simulink model "PID_PI_LADRC"  (R2021a)
settings: Solver=VariableStepAuto  StartTime=0.0  StopTime=Tsim  RelTol=1e-3
undefined symbols (not defined in the file or in its folder): Ac, Alpha, Bc, Cc, Cg, Kconva, Kconvp, Krad, L, mcecool, mcehot, mcerad, n, Rp, Tamb, Vfan, zo
libraries: pid_lib x1
settings Model: Creator=djah0  LastModifiedBy=djah0
settings DataIOCC: ReturnWorkspaceOutputs=off

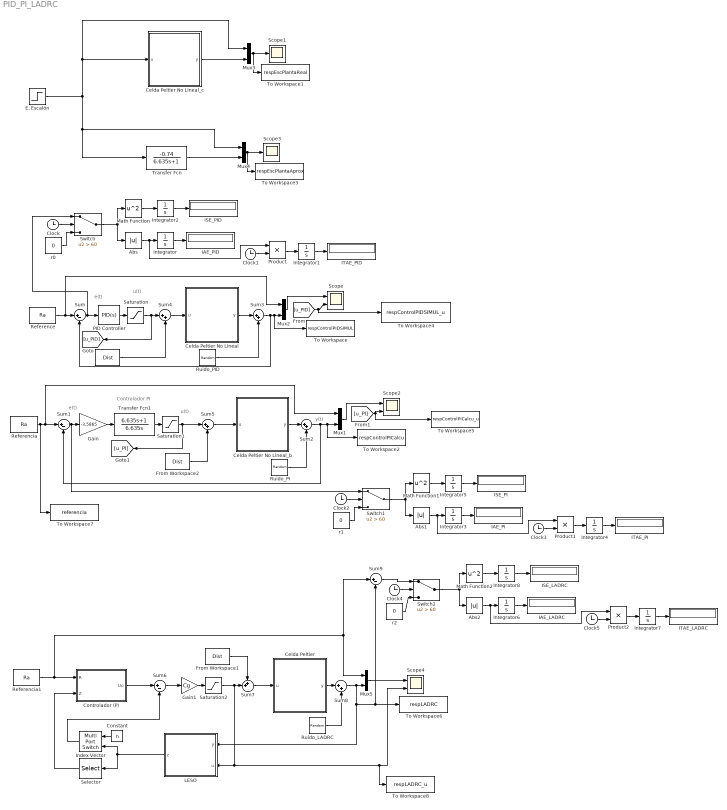
== system PID_PI_LADRC ==
  note: Controlador PI
  note: e(t)
  note: y(t)
  note: u(t)
  note: e(t)
  note: u(t)
  " " : FromWorkspace  VariableName=Dist
  Abs : Abs
  Abs1 : Abs
  Abs2 : Abs
  Celda Peltier : Subsystem
  Celda Peltier No Lineal : Subsystem
  Celda Peltier No Lineal_b : Subsystem
  Celda Peltier No Lineal_c : Subsystem
  Clock{,1..5} (6 alike) : Clock
  Constant : Constant  Value=n
  Controlador (P) : Subsystem
  E. Escalón : Step  Time=0  After=26  SampleTime=0
  From Workspace1 : FromWorkspace  VariableName=Dist
  From Workspace2 : FromWorkspace  VariableName=Dist
  Gain : Gain  Gain=-3.5865
  Gain1 : Gain  Gain=Cg
  IAE_LADRC : Display
  IAE_PI : Display
  IAE_PID : Display
  ISE_LADRC : Display
  ISE_PI : Display
  ISE_PID : Display
  ITAE_LADRC : Display
  ITAE_PI : Display
  ITAE_PID : Display
  Index Vector : MultiPortSwitch  Inputs=1
  Integrator{,1..8} (9 alike) : Integrator
  LESO : Subsystem
  Math Function : Math  Operator=square  SaturateOnIntegerOverflow=on
  Math Function1 : Math  Operator=square  SaturateOnIntegerOverflow=on
  Math Function2 : Math  Operator=square  SaturateOnIntegerOverflow=on
  Mux{1..5} (5 alike) : Mux  Inputs=2
  PID Controller : pid_lib/PID Controller  Controller=PID  Form=Parallel  TimeDomain=Continuous-time  UseExternalTs=off  SampleTime=-1  IntegratorMethod=Forward Euler  FilterMethod=Forward Euler  ControllerParametersSource=internal  P=-7.59310160847849  I=-3.05370465594005  D=0.689315335908169  UseFilter=on  N=11.0154253255872  TunerSelectOption=Transfer Function Based (PID Tuner App)  InitialConditionSource=internal  InitialConditionForIntegrator=26  InitialConditionForFilter=0  DifferentiatorICPrevScaledInput=0  ExternalReset=none  TrackingMode=off  Kt=1  LimitOutput=off  SatLimitsSource=internal  UpperSaturationLimit=inf  LowerSaturationLimit=-inf  LinearizeAsGain=on  AntiWindupMode=none  Kb=1  POutMin=[]  POutMax=[]  IOutMin=[]  IOutMax=[]  DOutMin=[]  DOutMax=[]  NOutMin=[]  NOutMax=[]  SumOutMin=[]  SumOutMax=[]  SaturationOutMin=[]  SaturationOutMax=[]  PParamMin=[]  PParamMax=[]  IParamMin=[]  IParamMax=[]  DParamMin=[]  DParamMax=[]  NParamMin=[]  NParamMax=[]  KbParamMin=[]  KbParamMax=[]  KtParamMin=[]  KtParamMax=[]  KbOutMin=[]  KbOutMax=[]  KtOutMin=[]  KtOutMax=[]  IntegratorOutMin=[]  IntegratorOutMax=[]  FilterOutMin=[]  FilterOutMax=[]  SumI1OutMin=[]  SumI1OutMax=[]  SumI2OutMin=[]  SumI2OutMax=[]  SumI3OutMin=[]  SumI3OutMax=[]  SumI4OutMin=[]  SumI4OutMax=[]  SumDOutMin=[]  SumDOutMax=[]  DifferentiatorOutMin=[]  DifferentiatorOutMax=[]  FilterDiffOutCoefMin=[]  FilterDiffOutCoefMax=[]  ReciprocalOutMin=[]  ReciprocalOutMax=[]  SumDenOutMin=[]  SumDenOutMax=[]  SumNumOutMin=[]  SumNumOutMax=[]  DivideOutMin=[]  DivideOutMax=[]  UdiffTsProdOutMin=[]  UdiffTsProdOutMax=[]  NTsProdOutMin=[]  NTsProdOutMax=[]  UintegralTsProdOutMin=[]  UintegralTsProdOutMax=[]  UngainTsProdOutMin=[]  UngainTsProdOutMax=[]  IntegratorContinuousStateAttributes=''  IntegratorStateMustResolveToSignalObject=off  IntegratorRTWStateStorageClass=Auto  FilterContinuousStateAttributes=''  FilterStateMustResolveToSignalObject=off  FilterRTWStateStorageClass=Auto  ParallelPVariant=InternalParameters  IdealPVariant=Disabled  IVariant=InternalParameters  DVariant=InternalParameters  IntegratorVariant=Continuous  SatVariant=Disabled  AWVariant=Passthrough  PCopyVariant=Disabled  TRVariant=Disabled  FdbkBlocksVariant=Forward  IdealPFdbkVariant=Disabled  SatFdbkVariant=Disabled  DerivativeFilterVariant=ContFilter  NVariant=InternalParameters  NCopyVariant=Disabled  FilterICVariant=InternalICsFilter  IntegratorICVariant=InternalICs  ExternalResetVariant=Disabled  TRSumVariant=Passthrough  SumFdbkVariant=Disabled  SumVariant=Sum_PID  TsampFilterVariant=InternalTs  TsampNgainVariant=Passthrough  TsampIntegralVariant=Passthrough  ExternalSaturationOutDataTypeStr=Inherit: Same as second input
  Product : Product
  Product1 : Product
  Product2 : Product
  Reference : FromWorkspace  VariableName=Ra
  Referencia : FromWorkspace  VariableName=Ra
  Referencia1 : FromWorkspace  VariableName=Ra
  Ruido_LADRC : RandomNumber  Variance=0.002  SampleTime=0.2
  Ruido_PI : RandomNumber  Variance=0.002  SampleTime=0.2
  Ruido_PID : RandomNumber  Variance=0.002  SampleTime=0.2
  Saturation : Saturate  UpperLimit=100  LowerLimit=0
  Saturation1 : Saturate  UpperLimit=100  LowerLimit=0
  Saturation2 : Saturate  UpperLimit=100  LowerLimit=0
  Scope : Scope  NumInputPorts=2
  Scope1 : Scope
  Scope2 : Scope  NumInputPorts=2
  Scope3 : Scope
  Scope4 : Scope  NumInputPorts=2
  Selector : Selector  InputPortWidth=n  IndexOptions=Index vector (dialog)  Indices=1:n-1  OutputSizes=1
  Sum{,1,6,9} (4 alike) : Sum  Inputs=|+-
  Sum{2..5,8} (5 alike) : Sum  Inputs=|++
  Sum7 : Sum  Inputs=++|
  Switch : Switch  Criteria=u2 > Threshold  Threshold=60
  Switch1 : Switch  Criteria=u2 > Threshold  Threshold=60
  Switch2 : Switch  Criteria=u2 > Threshold  Threshold=60
  To Workspace : ToWorkspace  VariableName=respControlPIDSIMUL  SaveFormat=Timeseries  SampleTime=-1
  To Workspace1 : ToWorkspace  VariableName=respEscPlantaReal  SaveFormat=Timeseries  SampleTime=-1
  To Workspace2 : ToWorkspace  VariableName=respControlPICalcu  SaveFormat=Timeseries  SampleTime=-1
  To Workspace3 : ToWorkspace  VariableName=respEscPlantaAprox  SaveFormat=Timeseries  SampleTime=-1
  To Workspace4 : ToWorkspace  VariableName=respControlPIDSIMUL_u  SaveFormat=Timeseries  SampleTime=-1
  To Workspace5 : ToWorkspace  VariableName=respControlPICalcu_u  SaveFormat=Timeseries  SampleTime=-1
  To Workspace6 : ToWorkspace  VariableName=respLADRC  SaveFormat=Timeseries  SampleTime=-1
  To Workspace7 : ToWorkspace  VariableName=referencia  SaveFormat=Timeseries  SampleTime=-1
  To Workspace8 : ToWorkspace  VariableName=respLADRC_u  SaveFormat=Timeseries  SampleTime=-1
  Transfer Fcn : TransferFcn  Numerator=[-0.74]  Denominator=[6.635 1]
  Transfer Fcn1 : TransferFcn  Numerator=[6.635 1]  Denominator=[6.635 0]
  r0 : Constant  Value=0
  r1 : Constant  Value=0
  r2 : Constant  Value=0
  wires:
  Mux2/1 -> Scope/1
  Reference/1 -> Mux2/1, Sum/1
  Referencia/1 -> To Workspace7/1, Mux1/1, Sum1/1
  Sum1/1 -> Switch1/1, Gain/1
  Mux1/1 -> Scope2/1
  Gain/1 -> Transfer Fcn1/1
  Sum/1 -> Switch/1, PID Controller/1
  Sum2/1 -> Sum1/2, To Workspace2/1, Mux1/2
  Sum3/1 -> Sum/2, To Workspace/1, Mux2/2
  [u_PID] -> To Workspace4/1, Scope/2
  [u_PI] -> To Workspace5/1, Scope2/2
  PID Controller/1 -> Saturation/1
  Transfer Fcn1/1 -> Saturation1/1
  Saturation1/1 -> Sum5/1, [u_PI]
  Saturation/1 -> [u_PID], Sum4/1
  Sum4/1 -> Celda Peltier No Lineal/1(u)
  " "/1 -> Sum4/2
  Celda Peltier No Lineal/1(y) -> Sum3/1
  Celda Peltier No Lineal_b/1(y) -> Sum2/1
  Sum5/1 -> Celda Peltier No Lineal_b/1(u)
  From Workspace2/1 -> Sum5/2
  Abs/1 -> Product/1, Integrator/1
  Integrator/1 -> IAE_PID/1
  r0/1 -> Switch/3
  Clock/1 -> Switch/2
  Switch/1 -> Math Function/1, Abs/1
  Math Function/1 -> Integrator2/1
  Integrator2/1 -> ISE_PID/1
  Clock1/1 -> Product/2
  Product/1 -> Integrator1/1
  Integrator1/1 -> ITAE_PID/1
  Integrator4/1 -> ITAE_PI/1
  Integrator5/1 -> ISE_PI/1
  Math Function1/1 -> Integrator5/1
  Clock2/1 -> Switch1/2
  Switch1/1 -> Math Function1/1, Abs1/1
  r1/1 -> Switch1/3
  Product1/1 -> Integrator4/1
  Abs1/1 -> Product1/1, Integrator3/1
  Clock3/1 -> Product1/2
  Integrator3/1 -> IAE_PI/1
  Sum9/1 -> Switch2/1
  Switch2/1 -> Math Function2/1, Abs2/1
  Sum6/1 -> Gain1/1
  Math Function2/1 -> Integrator8/1
  Integrator6/1 -> IAE_LADRC/1
  Clock5/1 -> Product2/2
  Abs2/1 -> Product2/1, Integrator6/1
  r2/1 -> Switch2/3
  Constant/1 -> Index Vector/1
  Integrator7/1 -> ITAE_LADRC/1
  Product2/1 -> Integrator7/1
  Sum7/1 -> Celda Peltier/1(u)
  Index Vector/1 -> Sum6/2
  Celda Peltier/1(y) -> Sum8/1
  Selector/1 -> Controlador (P)/2(Z)
  LESO/1(z) -> Index Vector/2, Selector/1
  From Workspace1/1 -> Sum7/1
  Mux5/1 -> Scope4/1
  Integrator8/1 -> ISE_LADRC/1
  Clock4/1 -> Switch2/2
  Saturation2/1 -> To Workspace8/1, Scope4/2, LESO/2(u), Sum7/2
  Sum8/1 -> Sum9/2, To Workspace6/1, LESO/1(y), Mux5/2
  Gain1/1 -> Saturation2/1
  Controlador (P)/1(Uo) -> Sum6/1
  Referencia1/1 -> Mux5/1, Sum9/1, Controlador (P)/1(R)
  E. Escalón/1 -> Mux4/1, Transfer Fcn/1, Celda Peltier No Lineal_c/1(u), Mux3/1
  Transfer Fcn/1 -> Mux4/2
  Celda Peltier No Lineal_c/1(y) -> Mux3/2
  Mux3/1 -> Scope1/1, To Workspace1/1
  Mux4/1 -> Scope3/1, To Workspace3/1
  Ruido_PID/1 -> Sum3/2
  Ruido_PI/1 -> Sum2/2
  Ruido_LADRC/1 -> Sum8/2

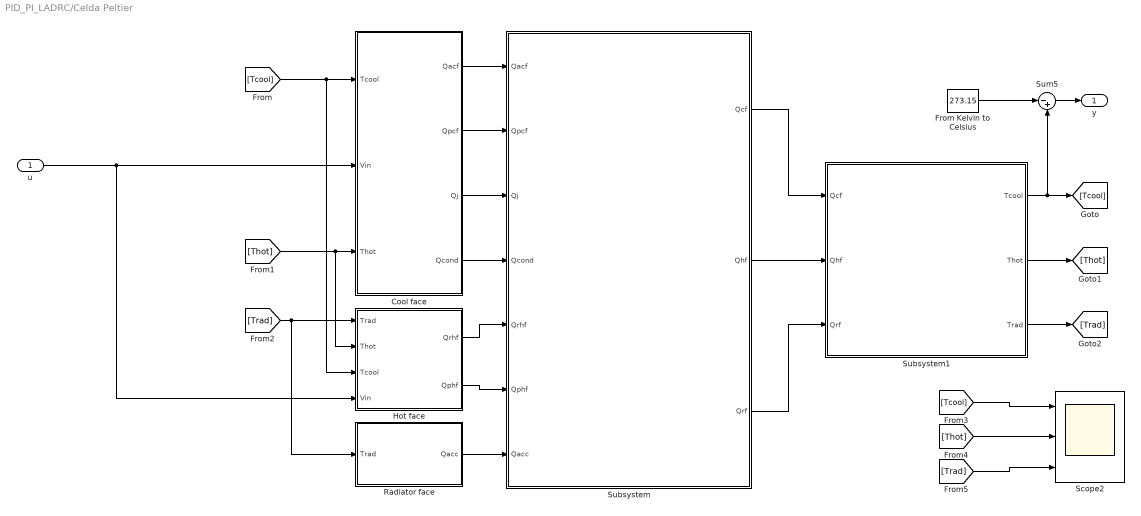
== system PID_PI_LADRC/Celda Peltier ==
  u : Inport
  Cool face : Subsystem
  From Kelvin to Celsius : Constant  Value=273.15
  Hot face : Subsystem
  Radiator face : Subsystem
  Scope2 : Scope  NumInputPorts=3
  Subsystem : Subsystem
  Subsystem1 : Subsystem
  Sum5 : Sum  Inputs=|-+
  y : Outport  VectorParamsAs1DForOutWhenUnconnected=off
  wires:
  u/1 -> Hot face/4(Vin), Cool face/2(Vin)
  [Tcool] -> Hot face/3(Tcool), Cool face/1(Tcool)
  Subsystem1/1(Tcool) -> [Tcool], Sum5/2
  Radiator face/1(Qacc) -> Subsystem/7(Qacc)
  Subsystem1/3(Trad) -> [Trad]
  [Thot] -> Hot face/2(Thot), Cool face/3(Thot)
  [Trad] -> Hot face/1(Trad), Radiator face/1(Trad)
  Subsystem1/2(Thot) -> [Thot]
  Cool face/2(Qpcf) -> Subsystem/2(Qpcf)
  Cool face/1(Qacf) -> Subsystem/1(Qacf)
  Cool face/3(Qj) -> Subsystem/3(Qj)
  Cool face/4(Qcond) -> Subsystem/4(Qcond)
  Subsystem/1(Qcf) -> Subsystem1/1(Qcf)
  Subsystem/2(Qhf) -> Subsystem1/2(Qhf)
  Subsystem/3(Qrf) -> Subsystem1/3(Qrf)
  Hot face/1(Qrhf) -> Subsystem/5(Qrhf)
  Hot face/2(Qphf) -> Subsystem/6(Qphf)
  Sum5/1 -> y/1
  From Kelvin to Celsius/1 -> Sum5/1
  [Tcool] -> Scope2/1
  [Thot] -> Scope2/2
  [Trad] -> Scope2/3

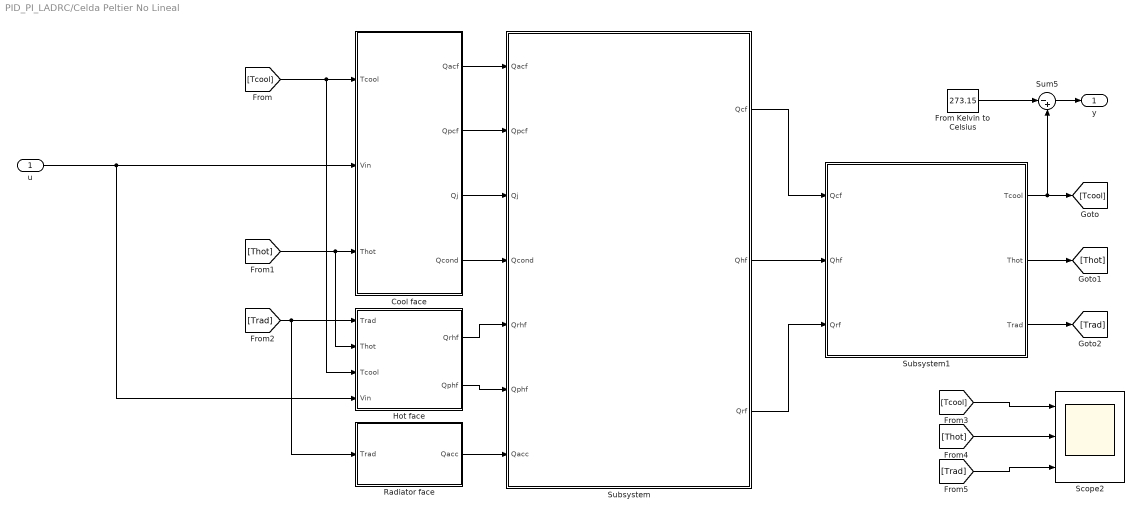
== system PID_PI_LADRC/Celda Peltier No Lineal ==
  u : Inport
  Cool face : Subsystem
  From Kelvin to Celsius : Constant  Value=273.15
  Hot face : Subsystem
  Radiator face : Subsystem
  Scope2 : Scope  NumInputPorts=3
  Subsystem : Subsystem
  Subsystem1 : Subsystem
  Sum5 : Sum  Inputs=|-+
  y : Outport  VectorParamsAs1DForOutWhenUnconnected=off
  wires:
  u/1 -> Hot face/4(Vin), Cool face/2(Vin)
  [Tcool] -> Hot face/3(Tcool), Cool face/1(Tcool)
  Subsystem1/1(Tcool) -> [Tcool], Sum5/2
  Radiator face/1(Qacc) -> Subsystem/7(Qacc)
  Subsystem1/3(Trad) -> [Trad]
  [Thot] -> Hot face/2(Thot), Cool face/3(Thot)
  [Trad] -> Hot face/1(Trad), Radiator face/1(Trad)
  Subsystem1/2(Thot) -> [Thot]
  Cool face/2(Qpcf) -> Subsystem/2(Qpcf)
  Cool face/1(Qacf) -> Subsystem/1(Qacf)
  Cool face/3(Qj) -> Subsystem/3(Qj)
  Cool face/4(Qcond) -> Subsystem/4(Qcond)
  Subsystem/1(Qcf) -> Subsystem1/1(Qcf)
  Subsystem/2(Qhf) -> Subsystem1/2(Qhf)
  Subsystem/3(Qrf) -> Subsystem1/3(Qrf)
  Hot face/1(Qrhf) -> Subsystem/5(Qrhf)
  Hot face/2(Qphf) -> Subsystem/6(Qphf)
  Sum5/1 -> y/1
  From Kelvin to Celsius/1 -> Sum5/1
  [Tcool] -> Scope2/1
  [Thot] -> Scope2/2
  [Trad] -> Scope2/3

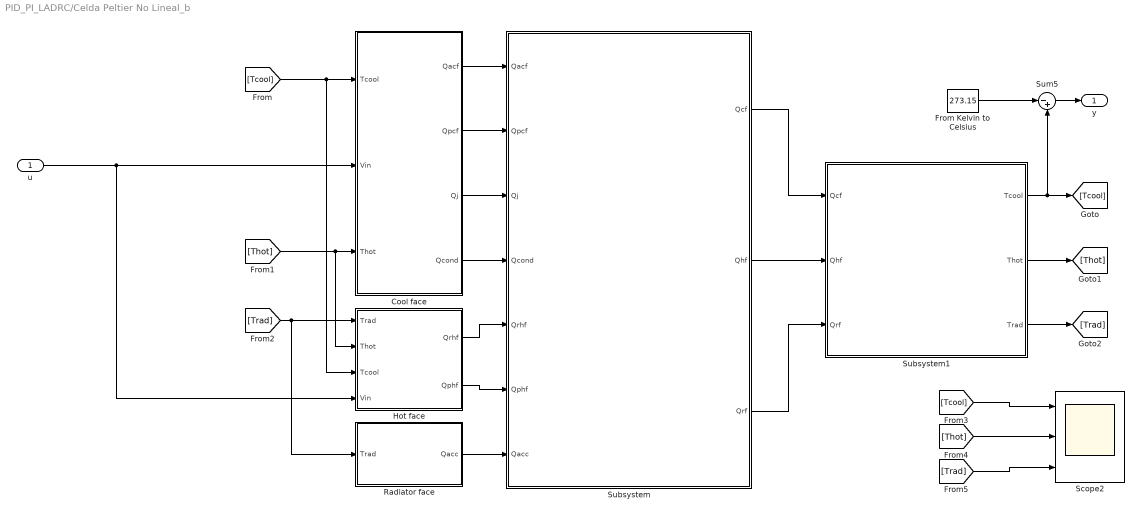
== system PID_PI_LADRC/Celda Peltier No Lineal_b ==
  u : Inport
  Cool face : Subsystem
  From Kelvin to Celsius : Constant  Value=273.15
  Hot face : Subsystem
  Radiator face : Subsystem
  Scope2 : Scope  NumInputPorts=3
  Subsystem : Subsystem
  Subsystem1 : Subsystem
  Sum5 : Sum  Inputs=|-+
  y : Outport  VectorParamsAs1DForOutWhenUnconnected=off
  wires:
  u/1 -> Hot face/4(Vin), Cool face/2(Vin)
  [Tcool] -> Hot face/3(Tcool), Cool face/1(Tcool)
  Subsystem1/1(Tcool) -> [Tcool], Sum5/2
  Radiator face/1(Qacc) -> Subsystem/7(Qacc)
  Subsystem1/3(Trad) -> [Trad]
  [Thot] -> Hot face/2(Thot), Cool face/3(Thot)
  [Trad] -> Hot face/1(Trad), Radiator face/1(Trad)
  Subsystem1/2(Thot) -> [Thot]
  Cool face/2(Qpcf) -> Subsystem/2(Qpcf)
  Cool face/1(Qacf) -> Subsystem/1(Qacf)
  Cool face/3(Qj) -> Subsystem/3(Qj)
  Cool face/4(Qcond) -> Subsystem/4(Qcond)
  Subsystem/1(Qcf) -> Subsystem1/1(Qcf)
  Subsystem/2(Qhf) -> Subsystem1/2(Qhf)
  Subsystem/3(Qrf) -> Subsystem1/3(Qrf)
  Hot face/1(Qrhf) -> Subsystem/5(Qrhf)
  Hot face/2(Qphf) -> Subsystem/6(Qphf)
  Sum5/1 -> y/1
  From Kelvin to Celsius/1 -> Sum5/1
  [Tcool] -> Scope2/1
  [Thot] -> Scope2/2
  [Trad] -> Scope2/3

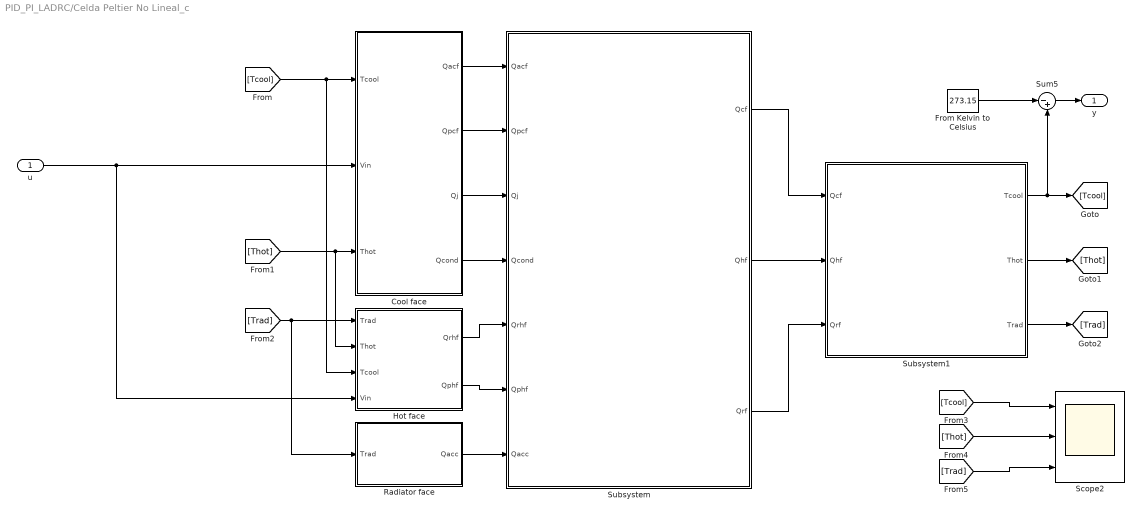
== system PID_PI_LADRC/Celda Peltier No Lineal_c ==
  u : Inport
  Cool face : Subsystem
  From Kelvin to Celsius : Constant  Value=273.15
  Hot face : Subsystem
  Radiator face : Subsystem
  Scope2 : Scope  NumInputPorts=3
  Subsystem : Subsystem
  Subsystem1 : Subsystem
  Sum5 : Sum  Inputs=|-+
  y : Outport  VectorParamsAs1DForOutWhenUnconnected=off
  wires:
  u/1 -> Hot face/4(Vin), Cool face/2(Vin)
  [Tcool] -> Hot face/3(Tcool), Cool face/1(Tcool)
  Subsystem1/1(Tcool) -> [Tcool], Sum5/2
  Radiator face/1(Qacc) -> Subsystem/7(Qacc)
  Subsystem1/3(Trad) -> [Trad]
  [Thot] -> Hot face/2(Thot), Cool face/3(Thot)
  [Trad] -> Hot face/1(Trad), Radiator face/1(Trad)
  Subsystem1/2(Thot) -> [Thot]
  Cool face/2(Qpcf) -> Subsystem/2(Qpcf)
  Cool face/1(Qacf) -> Subsystem/1(Qacf)
  Cool face/3(Qj) -> Subsystem/3(Qj)
  Cool face/4(Qcond) -> Subsystem/4(Qcond)
  Subsystem/1(Qcf) -> Subsystem1/1(Qcf)
  Subsystem/2(Qhf) -> Subsystem1/2(Qhf)
  Subsystem/3(Qrf) -> Subsystem1/3(Qrf)
  Hot face/1(Qrhf) -> Subsystem/5(Qrhf)
  Hot face/2(Qphf) -> Subsystem/6(Qphf)
  Sum5/1 -> y/1
  From Kelvin to Celsius/1 -> Sum5/1
  [Tcool] -> Scope2/1
  [Thot] -> Scope2/2
  [Trad] -> Scope2/3

== system PID_PI_LADRC/Controlador (P) ==
  R : Inport
  Z : Inport  Port=2
  Gain : Gain  Gain=0.5
  Sum1 : Sum  Inputs=-+|
  Uo : Outport  VectorParamsAs1DForOutWhenUnconnected=off
  wires:
  Gain/1 -> Uo/1
  Z/1 -> Sum1/1
  R/1 -> Sum1/2
  Sum1/1 -> Gain/1

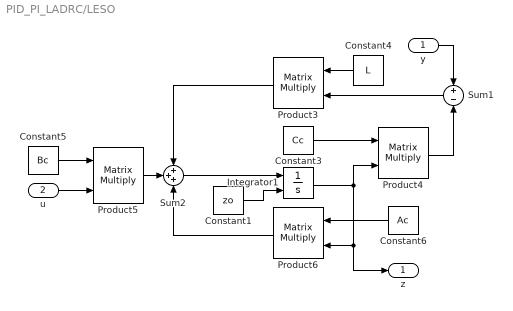
== system PID_PI_LADRC/LESO ==
  y : Inport
  u : Inport  Port=2
  Constant1 : Constant  Value=zo  VectorParams1D=off
  Constant3 : Constant  Value=Cc  VectorParams1D=off
  Constant4 : Constant  Value=L  VectorParams1D=off
  Constant5 : Constant  Value=Bc  VectorParams1D=off
  Constant6 : Constant  Value=Ac  VectorParams1D=off
  Integrator1 : Integrator  InitialConditionSource=external  InitialCondition=[Tamb;0]
  Product{3..6} (4 alike) : Product  Multiplication=Matrix(*)
  Sum1 : Sum  Inputs=+|-
  Sum2 : Sum  Inputs=+++
  z : Outport  VectorParamsAs1DForOutWhenUnconnected=off
  wires:
  Constant6/1 -> Product6/1
  Sum1/1 -> Product3/2
  Product6/1 -> Sum2/3
  Constant4/1 -> Product3/1
  Product4/1 -> Sum1/2
  Sum2/1 -> Integrator1/1
  Constant5/1 -> Product5/1
  Product5/1 -> Sum2/2
  Integrator1/1 -> Product4/2, z/1, Product6/2
  Constant3/1 -> Product4/1
  Product3/1 -> Sum2/1
  y/1 -> Sum1/1
  u/1 -> Product5/2
  Constant1/1 -> Integrator1/2

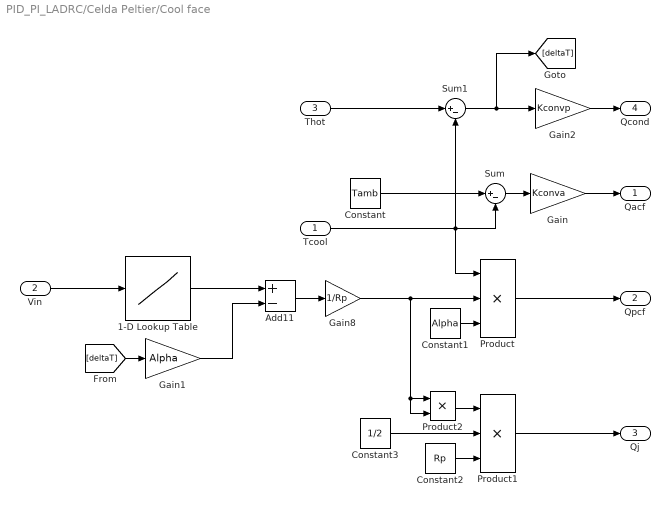
== system PID_PI_LADRC/Celda Peltier/Cool face ==
  Tcool : Inport
  Vin : Inport  Port=2
  Thot : Inport  Port=3
  1-D Lookup Table : Lookup_n-D  NumberOfTableDimensions=1  BreakpointsForDimension1=[0,10,20,30,40,100]  Table=[0,0.625,1.378,2.138,2.891,7.23]  RndMeth=Simplest  InputSameDT=on
  Add11 : Sum  Inputs=+-
  Constant : Constant  Value=Tamb
  Constant1 : Constant  Value=Alpha
  Constant2 : Constant  Value=Rp
  Constant3 : Constant  Value=1/2
  Gain : Gain  Gain=Kconva
  Gain1 : Gain  Gain=Alpha
  Gain2 : Gain  Gain=Kconvp
  Gain8 : Gain  Gain=1/Rp
  Product : Product  Inputs=3
  Product1 : Product  Inputs=3
  Product2 : Product
  Sum : Sum  Inputs=|+-
  Sum1 : Sum  Inputs=|+-
  Qacf : Outport  VectorParamsAs1DForOutWhenUnconnected=off
  Qpcf : Outport  Port=2  VectorParamsAs1DForOutWhenUnconnected=off
  Qj : Outport  Port=3  VectorParamsAs1DForOutWhenUnconnected=off
  Qcond : Outport  Port=4  VectorParamsAs1DForOutWhenUnconnected=off
  wires:
  Constant1/1 -> Product/3
  Sum1/1 -> Gain2/1, [deltaT]
  Sum/1 -> Gain/1
  Constant/1 -> Sum/1
  Product2/1 -> Product1/1
  Constant2/1 -> Product1/3
  Constant3/1 -> Product1/2
  Tcool/1 -> Sum1/2, Product/1, Sum/2
  Gain/1 -> Qacf/1
  Gain2/1 -> Qcond/1
  Product/1 -> Qpcf/1
  Product1/1 -> Qj/1
  Thot/1 -> Sum1/1
  Vin/1 -> 1-D Lookup Table/1
  Gain8/1 -> Product2/2, Product2/1, Product/2
  Add11/1 -> Gain8/1
  1-D Lookup Table/1 -> Add11/1
  [deltaT] -> Gain1/1
  Gain1/1 -> Add11/2

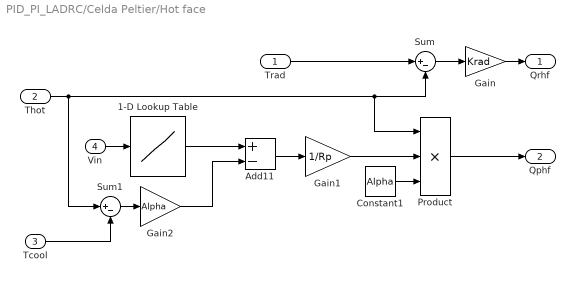
== system PID_PI_LADRC/Celda Peltier/Hot face ==
  Trad : Inport
  Thot : Inport  Port=2
  Tcool : Inport  Port=3
  Vin : Inport  Port=4
  1-D Lookup Table : Lookup_n-D  NumberOfTableDimensions=1  BreakpointsForDimension1=[0,10,20,30,40,100]  Table=[0,0.625,1.378,2.138,2.891,7.23]  RndMeth=Simplest  InputSameDT=on
  Add11 : Sum  Inputs=+-
  Constant1 : Constant  Value=Alpha
  Gain : Gain  Gain=Krad
  Gain1 : Gain  Gain=1/Rp
  Gain2 : Gain  Gain=Alpha
  Product : Product  Inputs=3
  Sum : Sum  Inputs=|+-
  Sum1 : Sum  Inputs=|+-
  Qrhf : Outport  VectorParamsAs1DForOutWhenUnconnected=off
  Qphf : Outport  Port=2  VectorParamsAs1DForOutWhenUnconnected=off
  wires:
  Sum/1 -> Gain/1
  Trad/1 -> Sum/1
  Gain/1 -> Qrhf/1
  Thot/1 -> Sum1/1, Product/1, Sum/2
  Product/1 -> Qphf/1
  Constant1/1 -> Product/3
  Add11/1 -> Gain1/1
  1-D Lookup Table/1 -> Add11/1
  Vin/1 -> 1-D Lookup Table/1
  Gain2/1 -> Add11/2
  Gain1/1 -> Product/2
  Sum1/1 -> Gain2/1
  Tcool/1 -> Sum1/2

== system PID_PI_LADRC/Celda Peltier/Radiator face ==
  Trad : Inport
  Constant : Constant  Value=Tamb
  Constant1 : Constant  Value=0.81
  Constant2 : Constant  Value=0.0032*(Vfan^3) - 0.24*(Vfan^2) + 6.6*Vfan - 56
  Constant3 : Constant  Value=Vfan
  Product : Product
  Sum : Sum  Inputs=+-|
  Switch : Switch  Criteria=u2 > Threshold  Threshold=22
  Qacc : Outport  VectorParamsAs1DForOutWhenUnconnected=off
  wires:
  Constant3/1 -> Switch/2
  Switch/1 -> Product/2
  Trad/1 -> Sum/2
  Sum/1 -> Product/1
  Product/1 -> Qacc/1
  Constant/1 -> Sum/1
  Constant2/1 -> Switch/1
  Constant1/1 -> Switch/3

== system PID_PI_LADRC/Celda Peltier/Subsystem ==
  Qacf : Inport
  Qpcf : Inport  Port=2
  Qj : Inport  Port=3
  Qcond : Inport  Port=4
  Qrhf : Inport  Port=5
  Qphf : Inport  Port=6
  Qacc : Inport  Port=7
  sum1 : Sum  Inputs=+--+
  sum2 : Sum  Inputs=+++-
  sum3 : Sum  Inputs=+-
  Qcf : Outport  VectorParamsAs1DForOutWhenUnconnected=off
  Qhf : Outport  Port=2  VectorParamsAs1DForOutWhenUnconnected=off
  Qrf : Outport  Port=3  VectorParamsAs1DForOutWhenUnconnected=off
  wires:
  Qcond/1 -> sum2/4, sum1/4
  Qj/1 -> sum2/3, sum1/3
  Qpcf/1 -> sum1/2
  Qacf/1 -> sum1/1
  Qrhf/1 -> sum3/2, sum2/1
  sum3/1 -> Qrf/1
  sum1/1 -> Qcf/1
  Qphf/1 -> sum2/2
  Qacc/1 -> sum3/1
  sum2/1 -> Qhf/1

== system PID_PI_LADRC/Celda Peltier/Subsystem1 ==
  Qcf : Inport
  Qhf : Inport  Port=2
  Qrf : Inport  Port=3
  Gain : Gain  Gain=1/mcecool
  Gain1 : Gain  Gain=1/mcehot
  Gain2 : Gain  Gain=1/mcerad
  Integrator : Integrator  InitialCondition=Tamb
  Integrator1 : Integrator  InitialCondition=Tamb
  Integrator2 : Integrator  InitialCondition=Tamb
  Tcool : Outport  VectorParamsAs1DForOutWhenUnconnected=off
  Thot : Outport  Port=2  VectorParamsAs1DForOutWhenUnconnected=off
  Trad : Outport  Port=3  VectorParamsAs1DForOutWhenUnconnected=off
  wires:
  Integrator1/1 -> Thot/1
  Gain2/1 -> Integrator2/1
  Gain1/1 -> Integrator1/1
  Qcf/1 -> Gain/1
  Integrator2/1 -> Trad/1
  Qhf/1 -> Gain1/1
  Gain/1 -> Integrator/1
  Integrator/1 -> Tcool/1
  Qrf/1 -> Gain2/1

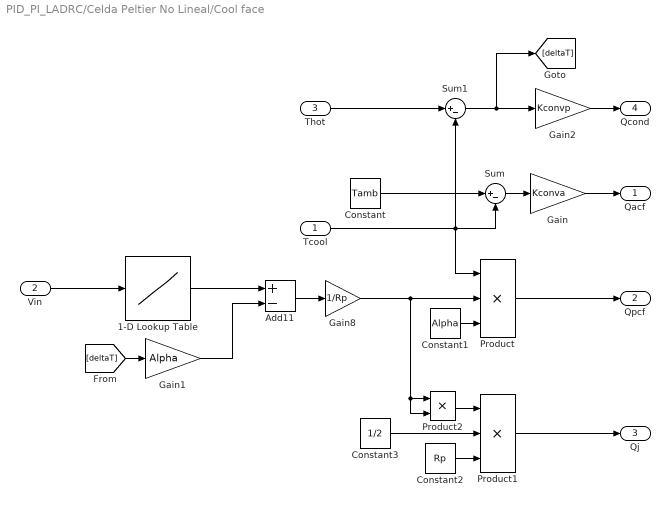
== system PID_PI_LADRC/Celda Peltier No Lineal/Cool face ==
  Tcool : Inport
  Vin : Inport  Port=2
  Thot : Inport  Port=3
  1-D Lookup Table : Lookup_n-D  NumberOfTableDimensions=1  BreakpointsForDimension1=[0,10,20,30,40,100]  Table=[0,0.625,1.378,2.138,2.891,7.23]  RndMeth=Simplest  InputSameDT=on
  Add11 : Sum  Inputs=+-
  Constant : Constant  Value=Tamb
  Constant1 : Constant  Value=Alpha
  Constant2 : Constant  Value=Rp
  Constant3 : Constant  Value=1/2
  Gain : Gain  Gain=Kconva
  Gain1 : Gain  Gain=Alpha
  Gain2 : Gain  Gain=Kconvp
  Gain8 : Gain  Gain=1/Rp
  Product : Product  Inputs=3
  Product1 : Product  Inputs=3
  Product2 : Product
  Sum : Sum  Inputs=|+-
  Sum1 : Sum  Inputs=|+-
  Qacf : Outport  VectorParamsAs1DForOutWhenUnconnected=off
  Qpcf : Outport  Port=2  VectorParamsAs1DForOutWhenUnconnected=off
  Qj : Outport  Port=3  VectorParamsAs1DForOutWhenUnconnected=off
  Qcond : Outport  Port=4  VectorParamsAs1DForOutWhenUnconnected=off
  wires:
  Constant1/1 -> Product/3
  Sum1/1 -> Gain2/1, [deltaT]
  Sum/1 -> Gain/1
  Constant/1 -> Sum/1
  Product2/1 -> Product1/1
  Constant2/1 -> Product1/3
  Constant3/1 -> Product1/2
  Tcool/1 -> Sum1/2, Product/1, Sum/2
  Gain/1 -> Qacf/1
  Gain2/1 -> Qcond/1
  Product/1 -> Qpcf/1
  Product1/1 -> Qj/1
  Thot/1 -> Sum1/1
  Vin/1 -> 1-D Lookup Table/1
  Gain8/1 -> Product2/2, Product2/1, Product/2
  Add11/1 -> Gain8/1
  1-D Lookup Table/1 -> Add11/1
  [deltaT] -> Gain1/1
  Gain1/1 -> Add11/2

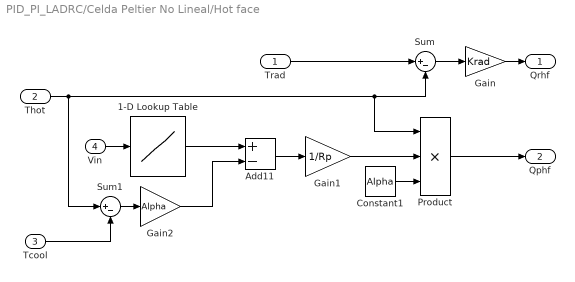
== system PID_PI_LADRC/Celda Peltier No Lineal/Hot face ==
  Trad : Inport
  Thot : Inport  Port=2
  Tcool : Inport  Port=3
  Vin : Inport  Port=4
  1-D Lookup Table : Lookup_n-D  NumberOfTableDimensions=1  BreakpointsForDimension1=[0,10,20,30,40,100]  Table=[0,0.625,1.378,2.138,2.891,7.23]  RndMeth=Simplest  InputSameDT=on
  Add11 : Sum  Inputs=+-
  Constant1 : Constant  Value=Alpha
  Gain : Gain  Gain=Krad
  Gain1 : Gain  Gain=1/Rp
  Gain2 : Gain  Gain=Alpha
  Product : Product  Inputs=3
  Sum : Sum  Inputs=|+-
  Sum1 : Sum  Inputs=|+-
  Qrhf : Outport  VectorParamsAs1DForOutWhenUnconnected=off
  Qphf : Outport  Port=2  VectorParamsAs1DForOutWhenUnconnected=off
  wires:
  Sum/1 -> Gain/1
  Trad/1 -> Sum/1
  Gain/1 -> Qrhf/1
  Thot/1 -> Sum1/1, Product/1, Sum/2
  Product/1 -> Qphf/1
  Constant1/1 -> Product/3
  Add11/1 -> Gain1/1
  1-D Lookup Table/1 -> Add11/1
  Vin/1 -> 1-D Lookup Table/1
  Gain2/1 -> Add11/2
  Gain1/1 -> Product/2
  Sum1/1 -> Gain2/1
  Tcool/1 -> Sum1/2

== system PID_PI_LADRC/Celda Peltier No Lineal/Radiator face ==
  Trad : Inport
  Constant : Constant  Value=Tamb
  Constant1 : Constant  Value=0.81
  Constant2 : Constant  Value=0.0032*(Vfan^3) - 0.24*(Vfan^2) + 6.6*Vfan - 56
  Constant3 : Constant  Value=Vfan
  Product : Product
  Sum : Sum  Inputs=+-|
  Switch : Switch  Criteria=u2 > Threshold  Threshold=22
  Qacc : Outport  VectorParamsAs1DForOutWhenUnconnected=off
  wires:
  Constant3/1 -> Switch/2
  Switch/1 -> Product/2
  Trad/1 -> Sum/2
  Sum/1 -> Product/1
  Product/1 -> Qacc/1
  Constant/1 -> Sum/1
  Constant2/1 -> Switch/1
  Constant1/1 -> Switch/3

== system PID_PI_LADRC/Celda Peltier No Lineal/Subsystem ==
  Qacf : Inport
  Qpcf : Inport  Port=2
  Qj : Inport  Port=3
  Qcond : Inport  Port=4
  Qrhf : Inport  Port=5
  Qphf : Inport  Port=6
  Qacc : Inport  Port=7
  sum1 : Sum  Inputs=+--+
  sum2 : Sum  Inputs=+++-
  sum3 : Sum  Inputs=+-
  Qcf : Outport  VectorParamsAs1DForOutWhenUnconnected=off
  Qhf : Outport  Port=2  VectorParamsAs1DForOutWhenUnconnected=off
  Qrf : Outport  Port=3  VectorParamsAs1DForOutWhenUnconnected=off
  wires:
  Qcond/1 -> sum2/4, sum1/4
  Qj/1 -> sum2/3, sum1/3
  Qpcf/1 -> sum1/2
  Qacf/1 -> sum1/1
  Qrhf/1 -> sum3/2, sum2/1
  sum3/1 -> Qrf/1
  sum1/1 -> Qcf/1
  Qphf/1 -> sum2/2
  Qacc/1 -> sum3/1
  sum2/1 -> Qhf/1

== system PID_PI_LADRC/Celda Peltier No Lineal/Subsystem1 ==
  Qcf : Inport
  Qhf : Inport  Port=2
  Qrf : Inport  Port=3
  Gain : Gain  Gain=1/mcecool
  Gain1 : Gain  Gain=1/mcehot
  Gain2 : Gain  Gain=1/mcerad
  Integrator : Integrator  InitialCondition=Tamb
  Integrator1 : Integrator  InitialCondition=Tamb
  Integrator2 : Integrator  InitialCondition=Tamb
  Tcool : Outport  VectorParamsAs1DForOutWhenUnconnected=off
  Thot : Outport  Port=2  VectorParamsAs1DForOutWhenUnconnected=off
  Trad : Outport  Port=3  VectorParamsAs1DForOutWhenUnconnected=off
  wires:
  Integrator1/1 -> Thot/1
  Gain2/1 -> Integrator2/1
  Gain1/1 -> Integrator1/1
  Qcf/1 -> Gain/1
  Integrator2/1 -> Trad/1
  Qhf/1 -> Gain1/1
  Gain/1 -> Integrator/1
  Integrator/1 -> Tcool/1
  Qrf/1 -> Gain2/1

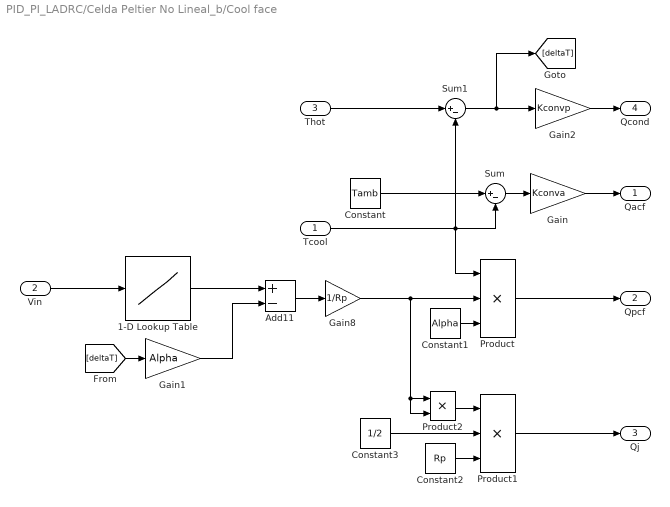
== system PID_PI_LADRC/Celda Peltier No Lineal_b/Cool face ==
  Tcool : Inport
  Vin : Inport  Port=2
  Thot : Inport  Port=3
  1-D Lookup Table : Lookup_n-D  NumberOfTableDimensions=1  BreakpointsForDimension1=[0,10,20,30,40,100]  Table=[0,0.625,1.378,2.138,2.891,7.23]  RndMeth=Simplest  InputSameDT=on
  Add11 : Sum  Inputs=+-
  Constant : Constant  Value=Tamb
  Constant1 : Constant  Value=Alpha
  Constant2 : Constant  Value=Rp
  Constant3 : Constant  Value=1/2
  Gain : Gain  Gain=Kconva
  Gain1 : Gain  Gain=Alpha
  Gain2 : Gain  Gain=Kconvp
  Gain8 : Gain  Gain=1/Rp
  Product : Product  Inputs=3
  Product1 : Product  Inputs=3
  Product2 : Product
  Sum : Sum  Inputs=|+-
  Sum1 : Sum  Inputs=|+-
  Qacf : Outport  VectorParamsAs1DForOutWhenUnconnected=off
  Qpcf : Outport  Port=2  VectorParamsAs1DForOutWhenUnconnected=off
  Qj : Outport  Port=3  VectorParamsAs1DForOutWhenUnconnected=off
  Qcond : Outport  Port=4  VectorParamsAs1DForOutWhenUnconnected=off
  wires:
  Constant1/1 -> Product/3
  Sum1/1 -> Gain2/1, [deltaT]
  Sum/1 -> Gain/1
  Constant/1 -> Sum/1
  Product2/1 -> Product1/1
  Constant2/1 -> Product1/3
  Constant3/1 -> Product1/2
  Tcool/1 -> Sum1/2, Product/1, Sum/2
  Gain/1 -> Qacf/1
  Gain2/1 -> Qcond/1
  Product/1 -> Qpcf/1
  Product1/1 -> Qj/1
  Thot/1 -> Sum1/1
  Vin/1 -> 1-D Lookup Table/1
  Gain8/1 -> Product2/2, Product2/1, Product/2
  Add11/1 -> Gain8/1
  1-D Lookup Table/1 -> Add11/1
  [deltaT] -> Gain1/1
  Gain1/1 -> Add11/2

== system PID_PI_LADRC/Celda Peltier No Lineal_b/Hot face ==
  Trad : Inport
  Thot : Inport  Port=2
  Tcool : Inport  Port=3
  Vin : Inport  Port=4
  1-D Lookup Table : Lookup_n-D  NumberOfTableDimensions=1  BreakpointsForDimension1=[0,10,20,30,40,100]  Table=[0,0.625,1.378,2.138,2.891,7.23]  RndMeth=Simplest  InputSameDT=on
  Add11 : Sum  Inputs=+-
  Constant1 : Constant  Value=Alpha
  Gain : Gain  Gain=Krad
  Gain1 : Gain  Gain=1/Rp
  Gain2 : Gain  Gain=Alpha
  Product : Product  Inputs=3
  Sum : Sum  Inputs=|+-
  Sum1 : Sum  Inputs=|+-
  Qrhf : Outport  VectorParamsAs1DForOutWhenUnconnected=off
  Qphf : Outport  Port=2  VectorParamsAs1DForOutWhenUnconnected=off
  wires:
  Sum/1 -> Gain/1
  Trad/1 -> Sum/1
  Gain/1 -> Qrhf/1
  Thot/1 -> Sum1/1, Product/1, Sum/2
  Product/1 -> Qphf/1
  Constant1/1 -> Product/3
  Add11/1 -> Gain1/1
  1-D Lookup Table/1 -> Add11/1
  Vin/1 -> 1-D Lookup Table/1
  Gain2/1 -> Add11/2
  Gain1/1 -> Product/2
  Sum1/1 -> Gain2/1
  Tcool/1 -> Sum1/2

== system PID_PI_LADRC/Celda Peltier No Lineal_b/Radiator face ==
  Trad : Inport
  Constant : Constant  Value=Tamb
  Constant1 : Constant  Value=0.81
  Constant2 : Constant  Value=0.0032*(Vfan^3) - 0.24*(Vfan^2) + 6.6*Vfan - 56
  Constant3 : Constant  Value=Vfan
  Product : Product
  Sum : Sum  Inputs=+-|
  Switch : Switch  Criteria=u2 > Threshold  Threshold=22
  Qacc : Outport  VectorParamsAs1DForOutWhenUnconnected=off
  wires:
  Constant3/1 -> Switch/2
  Switch/1 -> Product/2
  Trad/1 -> Sum/2
  Sum/1 -> Product/1
  Product/1 -> Qacc/1
  Constant/1 -> Sum/1
  Constant2/1 -> Switch/1
  Constant1/1 -> Switch/3

== system PID_PI_LADRC/Celda Peltier No Lineal_b/Subsystem ==
  Qacf : Inport
  Qpcf : Inport  Port=2
  Qj : Inport  Port=3
  Qcond : Inport  Port=4
  Qrhf : Inport  Port=5
  Qphf : Inport  Port=6
  Qacc : Inport  Port=7
  sum1 : Sum  Inputs=+--+
  sum2 : Sum  Inputs=+++-
  sum3 : Sum  Inputs=+-
  Qcf : Outport  VectorParamsAs1DForOutWhenUnconnected=off
  Qhf : Outport  Port=2  VectorParamsAs1DForOutWhenUnconnected=off
  Qrf : Outport  Port=3  VectorParamsAs1DForOutWhenUnconnected=off
  wires:
  Qcond/1 -> sum2/4, sum1/4
  Qj/1 -> sum2/3, sum1/3
  Qpcf/1 -> sum1/2
  Qacf/1 -> sum1/1
  Qrhf/1 -> sum3/2, sum2/1
  sum3/1 -> Qrf/1
  sum1/1 -> Qcf/1
  Qphf/1 -> sum2/2
  Qacc/1 -> sum3/1
  sum2/1 -> Qhf/1

== system PID_PI_LADRC/Celda Peltier No Lineal_b/Subsystem1 ==
  Qcf : Inport
  Qhf : Inport  Port=2
  Qrf : Inport  Port=3
  Gain : Gain  Gain=1/mcecool
  Gain1 : Gain  Gain=1/mcehot
  Gain2 : Gain  Gain=1/mcerad
  Integrator : Integrator  InitialCondition=Tamb
  Integrator1 : Integrator  InitialCondition=Tamb
  Integrator2 : Integrator  InitialCondition=Tamb
  Tcool : Outport  VectorParamsAs1DForOutWhenUnconnected=off
  Thot : Outport  Port=2  VectorParamsAs1DForOutWhenUnconnected=off
  Trad : Outport  Port=3  VectorParamsAs1DForOutWhenUnconnected=off
  wires:
  Integrator1/1 -> Thot/1
  Gain2/1 -> Integrator2/1
  Gain1/1 -> Integrator1/1
  Qcf/1 -> Gain/1
  Integrator2/1 -> Trad/1
  Qhf/1 -> Gain1/1
  Gain/1 -> Integrator/1
  Integrator/1 -> Tcool/1
  Qrf/1 -> Gain2/1

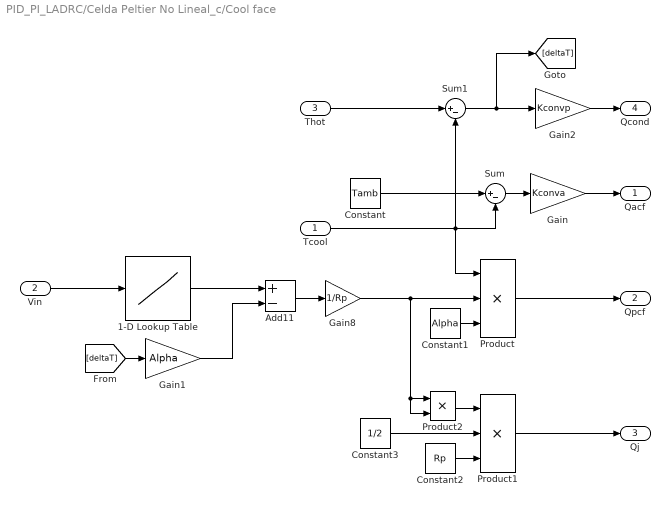
== system PID_PI_LADRC/Celda Peltier No Lineal_c/Cool face ==
  Tcool : Inport
  Vin : Inport  Port=2
  Thot : Inport  Port=3
  1-D Lookup Table : Lookup_n-D  NumberOfTableDimensions=1  BreakpointsForDimension1=[0,10,20,30,40,100]  Table=[0,0.625,1.378,2.138,2.891,7.23]  RndMeth=Simplest  InputSameDT=on
  Add11 : Sum  Inputs=+-
  Constant : Constant  Value=Tamb
  Constant1 : Constant  Value=Alpha
  Constant2 : Constant  Value=Rp
  Constant3 : Constant  Value=1/2
  Gain : Gain  Gain=Kconva
  Gain1 : Gain  Gain=Alpha
  Gain2 : Gain  Gain=Kconvp
  Gain8 : Gain  Gain=1/Rp
  Product : Product  Inputs=3
  Product1 : Product  Inputs=3
  Product2 : Product
  Sum : Sum  Inputs=|+-
  Sum1 : Sum  Inputs=|+-
  Qacf : Outport  VectorParamsAs1DForOutWhenUnconnected=off
  Qpcf : Outport  Port=2  VectorParamsAs1DForOutWhenUnconnected=off
  Qj : Outport  Port=3  VectorParamsAs1DForOutWhenUnconnected=off
  Qcond : Outport  Port=4  VectorParamsAs1DForOutWhenUnconnected=off
  wires:
  Constant1/1 -> Product/3
  Sum1/1 -> Gain2/1, [deltaT]
  Sum/1 -> Gain/1
  Constant/1 -> Sum/1
  Product2/1 -> Product1/1
  Constant2/1 -> Product1/3
  Constant3/1 -> Product1/2
  Tcool/1 -> Sum1/2, Product/1, Sum/2
  Gain/1 -> Qacf/1
  Gain2/1 -> Qcond/1
  Product/1 -> Qpcf/1
  Product1/1 -> Qj/1
  Thot/1 -> Sum1/1
  Vin/1 -> 1-D Lookup Table/1
  Gain8/1 -> Product2/2, Product2/1, Product/2
  Add11/1 -> Gain8/1
  1-D Lookup Table/1 -> Add11/1
  [deltaT] -> Gain1/1
  Gain1/1 -> Add11/2

== system PID_PI_LADRC/Celda Peltier No Lineal_c/Hot face ==
  Trad : Inport
  Thot : Inport  Port=2
  Tcool : Inport  Port=3
  Vin : Inport  Port=4
  1-D Lookup Table : Lookup_n-D  NumberOfTableDimensions=1  BreakpointsForDimension1=[0,10,20,30,40,100]  Table=[0,0.625,1.378,2.138,2.891,7.23]  RndMeth=Simplest  InputSameDT=on
  Add11 : Sum  Inputs=+-
  Constant1 : Constant  Value=Alpha
  Gain : Gain  Gain=Krad
  Gain1 : Gain  Gain=1/Rp
  Gain2 : Gain  Gain=Alpha
  Product : Product  Inputs=3
  Sum : Sum  Inputs=|+-
  Sum1 : Sum  Inputs=|+-
  Qrhf : Outport  VectorParamsAs1DForOutWhenUnconnected=off
  Qphf : Outport  Port=2  VectorParamsAs1DForOutWhenUnconnected=off
  wires:
  Sum/1 -> Gain/1
  Trad/1 -> Sum/1
  Gain/1 -> Qrhf/1
  Thot/1 -> Sum1/1, Product/1, Sum/2
  Product/1 -> Qphf/1
  Constant1/1 -> Product/3
  Add11/1 -> Gain1/1
  1-D Lookup Table/1 -> Add11/1
  Vin/1 -> 1-D Lookup Table/1
  Gain2/1 -> Add11/2
  Gain1/1 -> Product/2
  Sum1/1 -> Gain2/1
  Tcool/1 -> Sum1/2

== system PID_PI_LADRC/Celda Peltier No Lineal_c/Radiator face ==
  Trad : Inport
  Constant : Constant  Value=Tamb
  Constant1 : Constant  Value=0.81
  Constant2 : Constant  Value=0.0032*(Vfan^3) - 0.24*(Vfan^2) + 6.6*Vfan - 56
  Constant3 : Constant  Value=Vfan
  Product : Product
  Sum : Sum  Inputs=+-|
  Switch : Switch  Criteria=u2 > Threshold  Threshold=22
  Qacc : Outport  VectorParamsAs1DForOutWhenUnconnected=off
  wires:
  Constant3/1 -> Switch/2
  Switch/1 -> Product/2
  Trad/1 -> Sum/2
  Sum/1 -> Product/1
  Product/1 -> Qacc/1
  Constant/1 -> Sum/1
  Constant2/1 -> Switch/1
  Constant1/1 -> Switch/3

== system PID_PI_LADRC/Celda Peltier No Lineal_c/Subsystem ==
  Qacf : Inport
  Qpcf : Inport  Port=2
  Qj : Inport  Port=3
  Qcond : Inport  Port=4
  Qrhf : Inport  Port=5
  Qphf : Inport  Port=6
  Qacc : Inport  Port=7
  sum1 : Sum  Inputs=+--+
  sum2 : Sum  Inputs=+++-
  sum3 : Sum  Inputs=+-
  Qcf : Outport  VectorParamsAs1DForOutWhenUnconnected=off
  Qhf : Outport  Port=2  VectorParamsAs1DForOutWhenUnconnected=off
  Qrf : Outport  Port=3  VectorParamsAs1DForOutWhenUnconnected=off
  wires:
  Qcond/1 -> sum2/4, sum1/4
  Qj/1 -> sum2/3, sum1/3
  Qpcf/1 -> sum1/2
  Qacf/1 -> sum1/1
  Qrhf/1 -> sum3/2, sum2/1
  sum3/1 -> Qrf/1
  sum1/1 -> Qcf/1
  Qphf/1 -> sum2/2
  Qacc/1 -> sum3/1
  sum2/1 -> Qhf/1

== system PID_PI_LADRC/Celda Peltier No Lineal_c/Subsystem1 ==
  Qcf : Inport
  Qhf : Inport  Port=2
  Qrf : Inport  Port=3
  Gain : Gain  Gain=1/mcecool
  Gain1 : Gain  Gain=1/mcehot
  Gain2 : Gain  Gain=1/mcerad
  Integrator : Integrator  InitialCondition=Tamb
  Integrator1 : Integrator  InitialCondition=Tamb
  Integrator2 : Integrator  InitialCondition=Tamb
  Tcool : Outport  VectorParamsAs1DForOutWhenUnconnected=off
  Thot : Outport  Port=2  VectorParamsAs1DForOutWhenUnconnected=off
  Trad : Outport  Port=3  VectorParamsAs1DForOutWhenUnconnected=off
  wires:
  Integrator1/1 -> Thot/1
  Gain2/1 -> Integrator2/1
  Gain1/1 -> Integrator1/1
  Qcf/1 -> Gain/1
  Integrator2/1 -> Trad/1
  Qhf/1 -> Gain1/1
  Gain/1 -> Integrator/1
  Integrator/1 -> Tcool/1
  Qrf/1 -> Gain2/1
